simulink model "V511_L1_PIB"  (R2023b)
settings: Solver=VariableStepAuto  StartTime=0.0  StopTime=600  MaxStep=0.01  RelTol=1e-3
undefined symbols (not defined in the file): Kp
settings Model: Creator=td  LastModifiedBy=killer
settings SolverCC: AlgebraicLoopSolver=TrustRegion
settings DataIOCC: ReturnWorkspaceOutputs=off
settings OptimizationCC: ReuseModelBlockBuffer=off
settings DebuggingCC: UnconnectedInputMsg=warning  UnconnectedOutputMsg=warning  UnconnectedLineMsg=warning  ArithmeticOperatorsInVariantConditions=warning
settings ModelReferenceCC: EnableRefExpFcnMdlSchedulingChecks=on
settings SFSimCC: CustomCodeUndefinedFunction=UseInterfaceOnly

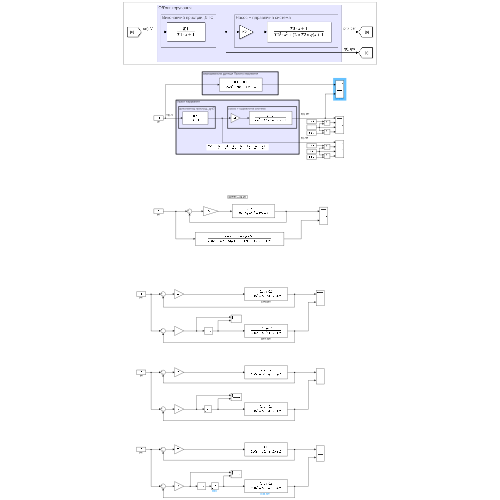
[thumbnail: Simulink's stored preview of the top-level diagram]
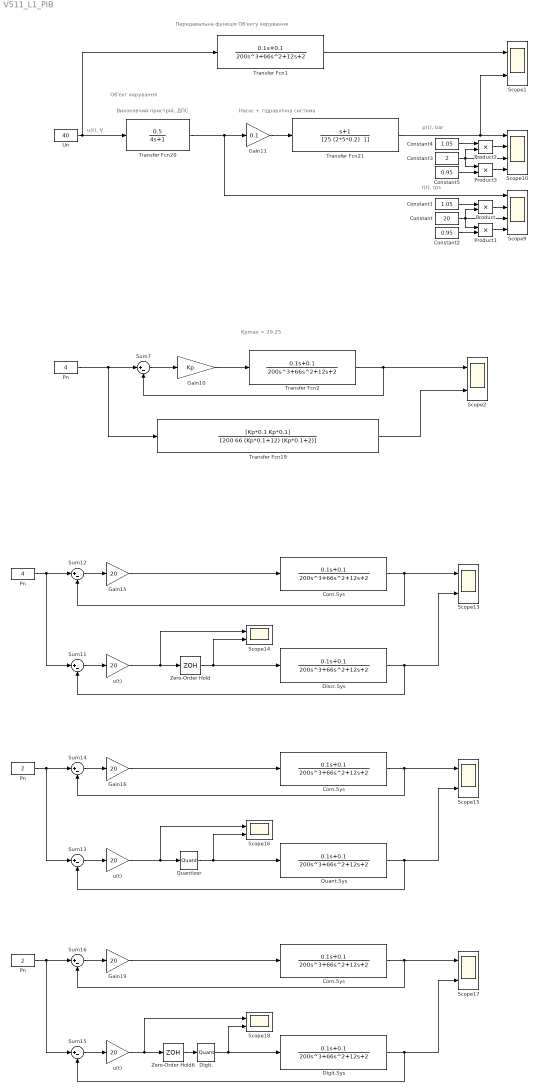
== system V511_L1_PIB ==
  note: Передавальна функція Об'єкту керування
  note: Kpmax = 29.25
  note: p(t), bar
  note: u(t), V
  note: Насос + гідравлічна система
  note: r(t), rps
  note: Виконавчий пристрій, ДПС
  note: Об'єкт керування
  " Pn" : Constant  Value=2
  " Pn " : Constant  Value=2
  " Quantizer " : Quantizer  QuantizationInterval=10
  " Zero-Order Hold " : ZeroOrderHold  SampleTime=0.1
  " u(t)   " : Gain  Gain=20
  Constant : Constant  Value=20
  Constant1 : Constant  Value=1.05
  Constant2 : Constant  Value=0.95
  Constant3 : Constant  Value=2
  Constant4 : Constant  Value=1.05
  Constant5 : Constant  Value=0.95
  Cont.Sys : TransferFcn  Numerator=[0.1 0.1]  Denominator=[200 66 12 2]
  "Cont.Sys  " : TransferFcn  Numerator=[0.1 0.1]  Denominator=[200 66 12 2]
  "Cont.Sys    " : TransferFcn  Numerator=[0.1 0.1]  Denominator=[200 66 12 2]
  Digit. : Quantizer  QuantizationInterval=2
  "Digit.Sys  " : TransferFcn  Numerator=[0.1 0.1]  Denominator=[200 66 12 2]
  Discr.Sys : TransferFcn  Numerator=[0.1 0.1]  Denominator=[200 66 12 2]
  Gain10 : Gain  Gain=Kp
  Gain11 : Gain  Gain=0.1
  Gain15 : Gain  Gain=20
  Gain16 : Gain  Gain=20
  Gain19 : Gain  Gain=20
  Pn : Constant  Value=4
  "Pn " : Constant  Value=4
  Product{,1..3} (4 alike) : Product
  Quant.Sys : TransferFcn  Numerator=[0.1 0.1]  Denominator=[200 66 12 2]
  Scope{1..2,13..18} (8 alike) : Scope  NumInputPorts=2
  Scope10 : Scope  NumInputPorts=4
  Scope9 : Scope  NumInputPorts=4
  Sum{7,11..16} (7 alike) : Sum  Inputs=|+-
  Transfer Fcn1 : TransferFcn  Numerator=[0.1 0.1]  Denominator=[200 66 12 2]
  Transfer Fcn19 : TransferFcn  Numerator=[Kp*0.1 Kp*0.1]  Denominator=[200 66 (Kp*0.1+12) (Kp*0.1+2)]
  Transfer Fcn2 : TransferFcn  Numerator=[0.1 0.1]  Denominator=[200 66 12 2]
  Transfer Fcn20 : TransferFcn  Numerator=[0.5]  Denominator=[4 1]
  Transfer Fcn21 : TransferFcn  Numerator=[1 1]  Denominator="[25 (2*5*0.2)  1]"
  Un : Constant  Value=40
  Zero-Order Hold6 : ZeroOrderHold  SampleTime=0.5
  u(t) : Gain  Gain=20
  "u(t) " : Gain  Gain=20
  wires:
  Un/1 -> Transfer Fcn1/1, Transfer Fcn20/1
  Constant5/1 -> Product3/2
  Product1/1 -> Scope9/4
  Product3/1 -> Scope10/4
  Transfer Fcn20/1 -> Scope9/1, Gain11/1
  Constant4/1 -> Product2/1
  Constant3/1 -> Product2/2, Product3/1, Scope10/3
  Product2/1 -> Scope10/2
  Gain11/1 -> Transfer Fcn21/1
  Transfer Fcn21/1 -> Scope1/2, Scope10/1
  Product/1 -> Scope9/2
  Constant2/1 -> Product1/2
  Constant/1 -> Product/2, Product1/1, Scope9/3
  Constant1/1 -> Product/1
  Transfer Fcn1/1 -> Scope1/1
  Gain10/1 -> Transfer Fcn2/1
  Pn/1 -> Transfer Fcn19/1, Sum7/1
  Transfer Fcn2/1 -> Scope2/1, Sum7/2
  Transfer Fcn19/1 -> Scope2/2
  Sum7/1 -> Gain10/1
  Sum13/1 -> "u(t) "/1
  "Pn "/1 -> Sum11/1, Sum12/1
  " Quantizer "/1 -> Quant.Sys/1, Scope16/2
  "Cont.Sys  "/1 -> Scope15/1, Sum14/2
  Sum15/1 -> " u(t)   "/1
  Gain19/1 -> "Cont.Sys    "/1
  "Digit.Sys  "/1 -> Scope17/2, Sum15/2
  " Pn "/1 -> Sum15/1, Sum16/1
  Digit./1 -> "Digit.Sys  "/1, Scope18/2
  u(t)/1 -> Scope14/1, " Zero-Order Hold "/1
  Sum16/1 -> Gain19/1
  Gain15/1 -> Cont.Sys/1
  " Pn"/1 -> Sum13/1, Sum14/1
  " Zero-Order Hold "/1 -> Discr.Sys/1, Scope14/2
  Zero-Order Hold6/1 -> Digit./1
  Gain16/1 -> "Cont.Sys  "/1
  Cont.Sys/1 -> Scope13/1, Sum12/2
  "Cont.Sys    "/1 -> Scope17/1, Sum16/2
  " u(t)   "/1 -> Zero-Order Hold6/1, Scope18/1
  Sum12/1 -> Gain15/1
  "u(t) "/1 -> " Quantizer "/1, Scope16/1
  Quant.Sys/1 -> Scope15/2, Sum13/2
  Sum11/1 -> u(t)/1
  Sum14/1 -> Gain16/1
  Discr.Sys/1 -> Scope13/2, Sum11/2
